simulink model "ng_pv_dynamic_dbus_p_4_ss_pmu"  (Simulink 8.8)
settings: Solver=ode4  StartTime=0.0  StopTime=inf  FixedStep=0.000125  RelTol=1e-3  EnableMultiTasking=on
PreLoadFcn:
  | Ts=125e-6;Core_Num = 0; np=1; nq=1; Vmin=.9;
PostLoadFcn:
  | Ts=125e-6;Core_Num = 0; np=1; nq=1; Vmin=.9;
InitFcn:
  | Ts=125e-6;Core_Num = 0; np=1; nq=1; Vmin=.9;
libraries: powerlib_meascontrol x180, rtio_generic_c37_118 x22, simulink x22, opal_lib x4, artemis x1, rtlab x1, powerlib x1
(part 2 of 4)

== system ng_pv_dynamic_dbus_p_4_ss_pmu/SS_PMU/Subsystem31 ==
  PMU in : Inport
  Bus Selector : BusSelector  OutputSignals=Measurements,FREQ,FROC
  Constant28 : Constant  Value=-1
  Constant29 : Constant  Value=-1
  Subsystem : Subsystem
  Phasors : Outport
  Analog : Outport  Port=2
  Ditigal : Outport  Port=3
  FREQ : Outport  Port=4
  FROC : Outport  Port=5
  wires:
  Subsystem/1(Out1) -> Bus Selector/1
  Bus Selector/1 -> Phasors/1  "<Measurements>"
  PMU in/1 -> Subsystem/1(In1)
  Constant28/1 -> Analog/1
  Constant29/1 -> Ditigal/1
  Bus Selector/2 -> FREQ/1  "<FREQ>"
  Bus Selector/3 -> FROC/1  "<FROC>"

== system ng_pv_dynamic_dbus_p_4_ss_pmu/SS_PMU/Subsystem32 ==
  PMU in : Inport
  Bus Selector : BusSelector  OutputSignals=Measurements,FREQ,FROC
  Constant28 : Constant  Value=-1
  Constant29 : Constant  Value=-1
  Subsystem : Subsystem
  Phasors : Outport
  Analog : Outport  Port=2
  Ditigal : Outport  Port=3
  FREQ : Outport  Port=4
  FROC : Outport  Port=5
  wires:
  Subsystem/1(Out1) -> Bus Selector/1
  Bus Selector/1 -> Phasors/1  "<Measurements>"
  PMU in/1 -> Subsystem/1(In1)
  Constant28/1 -> Analog/1
  Constant29/1 -> Ditigal/1
  Bus Selector/2 -> FREQ/1  "<FREQ>"
  Bus Selector/3 -> FROC/1  "<FROC>"

== system ng_pv_dynamic_dbus_p_4_ss_pmu/SS_PMU/Subsystem33 ==
  PMU in : Inport
  Bus Selector : BusSelector  OutputSignals=Measurements,FREQ,FROC
  Constant28 : Constant  Value=-1
  Constant29 : Constant  Value=-1
  Subsystem : Subsystem
  Phasors : Outport
  Analog : Outport  Port=2
  Ditigal : Outport  Port=3
  FREQ : Outport  Port=4
  FROC : Outport  Port=5
  wires:
  Subsystem/1(Out1) -> Bus Selector/1
  Bus Selector/1 -> Phasors/1  "<Measurements>"
  PMU in/1 -> Subsystem/1(In1)
  Constant28/1 -> Analog/1
  Constant29/1 -> Ditigal/1
  Bus Selector/2 -> FREQ/1  "<FREQ>"
  Bus Selector/3 -> FROC/1  "<FROC>"

== system ng_pv_dynamic_dbus_p_4_ss_pmu/SS_PMU/Subsystem34 ==
  PMU in : Inport
  Bus Selector : BusSelector  OutputSignals=Measurements,FREQ,FROC
  Constant28 : Constant  Value=-1
  Constant29 : Constant  Value=-1
  Subsystem : Subsystem
  Phasors : Outport
  Analog : Outport  Port=2
  Ditigal : Outport  Port=3
  FREQ : Outport  Port=4
  FROC : Outport  Port=5
  wires:
  Subsystem/1(Out1) -> Bus Selector/1
  Bus Selector/1 -> Phasors/1  "<Measurements>"
  PMU in/1 -> Subsystem/1(In1)
  Constant28/1 -> Analog/1
  Constant29/1 -> Ditigal/1
  Bus Selector/2 -> FREQ/1  "<FREQ>"
  Bus Selector/3 -> FROC/1  "<FROC>"

== system ng_pv_dynamic_dbus_p_4_ss_pmu/SS_PMU/Subsystem35 ==
  PMU in : Inport
  Bus Selector : BusSelector  OutputSignals=Measurements,FREQ,FROC
  Constant28 : Constant  Value=-1
  Constant29 : Constant  Value=-1
  Subsystem : Subsystem
  Phasors : Outport
  Analog : Outport  Port=2
  Ditigal : Outport  Port=3
  FREQ : Outport  Port=4
  FROC : Outport  Port=5
  wires:
  Subsystem/1(Out1) -> Bus Selector/1
  Bus Selector/1 -> Phasors/1  "<Measurements>"
  PMU in/1 -> Subsystem/1(In1)
  Constant28/1 -> Analog/1
  Constant29/1 -> Ditigal/1
  Bus Selector/2 -> FREQ/1  "<FREQ>"
  Bus Selector/3 -> FROC/1  "<FROC>"

== system ng_pv_dynamic_dbus_p_4_ss_pmu/SS_PMU/Subsystem36 ==
  PMU in : Inport
  Bus Selector : BusSelector  OutputSignals=Measurements,FREQ,FROC
  Constant28 : Constant  Value=-1
  Constant29 : Constant  Value=-1
  Subsystem : Subsystem
  Phasors : Outport
  Analog : Outport  Port=2
  Ditigal : Outport  Port=3
  FREQ : Outport  Port=4
  FROC : Outport  Port=5
  wires:
  Subsystem/1(Out1) -> Bus Selector/1
  Bus Selector/1 -> Phasors/1  "<Measurements>"
  PMU in/1 -> Subsystem/1(In1)
  Constant28/1 -> Analog/1
  Constant29/1 -> Ditigal/1
  Bus Selector/2 -> FREQ/1  "<FREQ>"
  Bus Selector/3 -> FROC/1  "<FROC>"

== system ng_pv_dynamic_dbus_p_4_ss_pmu/SS_PMU/Subsystem37 ==
  PMU in : Inport
  Bus Selector : BusSelector  OutputSignals=Measurements,FREQ,FROC
  Constant28 : Constant  Value=-1
  Constant29 : Constant  Value=-1
  Subsystem : Subsystem
  Phasors : Outport
  Analog : Outport  Port=2
  Ditigal : Outport  Port=3
  FREQ : Outport  Port=4
  FROC : Outport  Port=5
  wires:
  Subsystem/1(Out1) -> Bus Selector/1
  Bus Selector/1 -> Phasors/1  "<Measurements>"
  PMU in/1 -> Subsystem/1(In1)
  Constant28/1 -> Analog/1
  Constant29/1 -> Ditigal/1
  Bus Selector/2 -> FREQ/1  "<FREQ>"
  Bus Selector/3 -> FROC/1  "<FROC>"

== system ng_pv_dynamic_dbus_p_4_ss_pmu/SS_PMU/Subsystem38 ==
  PMU in : Inport
  Bus Selector : BusSelector  OutputSignals=Measurements,FREQ,FROC
  Constant28 : Constant  Value=-1
  Constant29 : Constant  Value=-1
  Subsystem : Subsystem
  Phasors : Outport
  Analog : Outport  Port=2
  Ditigal : Outport  Port=3
  FREQ : Outport  Port=4
  FROC : Outport  Port=5
  wires:
  Subsystem/1(Out1) -> Bus Selector/1
  Bus Selector/1 -> Phasors/1  "<Measurements>"
  PMU in/1 -> Subsystem/1(In1)
  Constant28/1 -> Analog/1
  Constant29/1 -> Ditigal/1
  Bus Selector/2 -> FREQ/1  "<FREQ>"
  Bus Selector/3 -> FROC/1  "<FROC>"

== system ng_pv_dynamic_dbus_p_4_ss_pmu/SS_PMU/Subsystem39 ==
  PMU in : Inport
  Bus Selector : BusSelector  OutputSignals=Measurements,FREQ,FROC
  Constant28 : Constant  Value=-1
  Constant29 : Constant  Value=-1
  Subsystem : Subsystem
  Phasors : Outport
  Analog : Outport  Port=2
  Ditigal : Outport  Port=3
  FREQ : Outport  Port=4
  FROC : Outport  Port=5
  wires:
  Subsystem/1(Out1) -> Bus Selector/1
  Bus Selector/1 -> Phasors/1  "<Measurements>"
  PMU in/1 -> Subsystem/1(In1)
  Constant28/1 -> Analog/1
  Constant29/1 -> Ditigal/1
  Bus Selector/2 -> FREQ/1  "<FREQ>"
  Bus Selector/3 -> FROC/1  "<FROC>"

== system ng_pv_dynamic_dbus_p_4_ss_pmu/SS_PMU/Subsystem4 ==
  Measurements : Inport
  Demux7 : Demux  Outputs=6
  Demux8 : Demux  Outputs=6
  Mux5 : Mux  Inputs=12
  Subsystem : Subsystem
  Phasors : Outport
  Phasor_Freq : Outport  Port=2
  FROC : Outport  Port=3
  wires:
  Mux5/1 -> Phasors/1
  Demux7/4 -> [Phase_Va]
  Demux7/1 -> [Mag_Va]
  Demux7/2 -> [Mag_Vb]
  Demux7/3 -> [Mag_Vc]
  Subsystem/1(Phasors_Vabc) -> Demux7/1
  Demux7/6 -> [Phase_Vc]
  Demux7/5 -> [Phase_Vb]
  Subsystem/3(Phasor_Freq) -> Phasor_Freq/1
  Measurements/1 -> Subsystem/1(Measurements1)
  Subsystem/4(Phasor_DTFreq) -> FROC/1
  Demux8/2 -> [Mag_Ib]
  Demux8/4 -> [Phase_Ia]
  Demux8/5 -> [Phase_Ib]
  Subsystem/2(Phasors_Iabc) -> Demux8/1
  Demux8/3 -> [Mag_Ic]
  Demux8/1 -> [Mag_Ia]
  Demux8/6 -> [Phase_Ic]
  [Phase_Ic] -> Mux5/12
  [Mag_Ic] -> Mux5/11
  [Phase_Ib] -> Mux5/10
  [Mag_Ib] -> Mux5/9
  [Phase_Ia] -> Mux5/8
  [Mag_Ia] -> Mux5/7
  [Phase_Vc] -> Mux5/6
  [Mag_Vc] -> Mux5/5
  [Phase_Vb] -> Mux5/4
  [Mag_Vb] -> Mux5/3
  [Phase_Va] -> Mux5/2
  [Mag_Va] -> Mux5/1

== system ng_pv_dynamic_dbus_p_4_ss_pmu/SS_PMU/Subsystem40 ==
  PMU in : Inport
  Bus Selector : BusSelector  OutputSignals=Measurements,FREQ,FROC
  Constant28 : Constant  Value=-1
  Constant29 : Constant  Value=-1
  Subsystem : Subsystem
  Phasors : Outport
  Analog : Outport  Port=2
  Ditigal : Outport  Port=3
  FREQ : Outport  Port=4
  FROC : Outport  Port=5
  wires:
  Subsystem/1(Out1) -> Bus Selector/1
  Bus Selector/1 -> Phasors/1  "<Measurements>"
  PMU in/1 -> Subsystem/1(In1)
  Constant28/1 -> Analog/1
  Constant29/1 -> Ditigal/1
  Bus Selector/2 -> FREQ/1  "<FREQ>"
  Bus Selector/3 -> FROC/1  "<FROC>"

== system ng_pv_dynamic_dbus_p_4_ss_pmu/SS_PMU/Subsystem41 ==
  PMU in : Inport
  Bus Selector : BusSelector  OutputSignals=Measurements,FREQ,FROC
  Constant28 : Constant  Value=-1
  Constant29 : Constant  Value=-1
  Subsystem : Subsystem
  Phasors : Outport
  Analog : Outport  Port=2
  Ditigal : Outport  Port=3
  FREQ : Outport  Port=4
  FROC : Outport  Port=5
  wires:
  Subsystem/1(Out1) -> Bus Selector/1
  Bus Selector/1 -> Phasors/1  "<Measurements>"
  PMU in/1 -> Subsystem/1(In1)
  Constant28/1 -> Analog/1
  Constant29/1 -> Ditigal/1
  Bus Selector/2 -> FREQ/1  "<FREQ>"
  Bus Selector/3 -> FROC/1  "<FROC>"

== system ng_pv_dynamic_dbus_p_4_ss_pmu/SS_PMU/Subsystem42 ==
  PMU in : Inport
  Bus Selector : BusSelector  OutputSignals=Measurements,FREQ,FROC
  Constant28 : Constant  Value=-1
  Constant29 : Constant  Value=-1
  Subsystem : Subsystem
  Phasors : Outport
  Analog : Outport  Port=2
  Ditigal : Outport  Port=3
  FREQ : Outport  Port=4
  FROC : Outport  Port=5
  wires:
  Subsystem/1(Out1) -> Bus Selector/1
  Bus Selector/1 -> Phasors/1  "<Measurements>"
  PMU in/1 -> Subsystem/1(In1)
  Constant28/1 -> Analog/1
  Constant29/1 -> Ditigal/1
  Bus Selector/2 -> FREQ/1  "<FREQ>"
  Bus Selector/3 -> FROC/1  "<FROC>"

== system ng_pv_dynamic_dbus_p_4_ss_pmu/SS_PMU/Subsystem43 ==
  PMU in : Inport
  Bus Selector : BusSelector  OutputSignals=Measurements,FREQ,FROC
  Constant28 : Constant  Value=-1
  Constant29 : Constant  Value=-1
  Subsystem : Subsystem
  Phasors : Outport
  Analog : Outport  Port=2
  Ditigal : Outport  Port=3
  FREQ : Outport  Port=4
  FROC : Outport  Port=5
  wires:
  Subsystem/1(Out1) -> Bus Selector/1
  Bus Selector/1 -> Phasors/1  "<Measurements>"
  PMU in/1 -> Subsystem/1(In1)
  Constant28/1 -> Analog/1
  Constant29/1 -> Ditigal/1
  Bus Selector/2 -> FREQ/1  "<FREQ>"
  Bus Selector/3 -> FROC/1  "<FROC>"

== system ng_pv_dynamic_dbus_p_4_ss_pmu/SS_PMU/Subsystem44 ==
  PMU in : Inport
  Bus Selector : BusSelector  OutputSignals=Measurements,FREQ,FROC
  Constant28 : Constant  Value=-1
  Constant29 : Constant  Value=-1
  Subsystem : Subsystem
  Phasors : Outport
  Analog : Outport  Port=2
  Ditigal : Outport  Port=3
  FREQ : Outport  Port=4
  FROC : Outport  Port=5
  wires:
  Subsystem/1(Out1) -> Bus Selector/1
  Bus Selector/1 -> Phasors/1  "<Measurements>"
  PMU in/1 -> Subsystem/1(In1)
  Constant28/1 -> Analog/1
  Constant29/1 -> Ditigal/1
  Bus Selector/2 -> FREQ/1  "<FREQ>"
  Bus Selector/3 -> FROC/1  "<FROC>"

== system ng_pv_dynamic_dbus_p_4_ss_pmu/SS_PMU/Subsystem5 ==
  Measurements : Inport
  Demux7 : Demux  Outputs=6
  Demux8 : Demux  Outputs=6
  Mux5 : Mux  Inputs=12
  Subsystem : Subsystem
  Phasors : Outport
  Phasor_Freq : Outport  Port=2
  FROC : Outport  Port=3
  wires:
  Mux5/1 -> Phasors/1
  Demux7/4 -> [Phase_Va]
  Demux7/1 -> [Mag_Va]
  Demux7/2 -> [Mag_Vb]
  Demux7/3 -> [Mag_Vc]
  Subsystem/1(Phasors_Vabc) -> Demux7/1
  Demux7/6 -> [Phase_Vc]
  Demux7/5 -> [Phase_Vb]
  Subsystem/3(Phasor_Freq) -> Phasor_Freq/1
  Measurements/1 -> Subsystem/1(Measurements1)
  Subsystem/4(Phasor_DTFreq) -> FROC/1
  Demux8/2 -> [Mag_Ib]
  Demux8/4 -> [Phase_Ia]
  Demux8/5 -> [Phase_Ib]
  Subsystem/2(Phasors_Iabc) -> Demux8/1
  Demux8/3 -> [Mag_Ic]
  Demux8/1 -> [Mag_Ia]
  Demux8/6 -> [Phase_Ic]
  [Phase_Ic] -> Mux5/12
  [Mag_Ic] -> Mux5/11
  [Phase_Ib] -> Mux5/10
  [Mag_Ib] -> Mux5/9
  [Phase_Ia] -> Mux5/8
  [Mag_Ia] -> Mux5/7
  [Phase_Vc] -> Mux5/6
  [Mag_Vc] -> Mux5/5
  [Phase_Vb] -> Mux5/4
  [Mag_Vb] -> Mux5/3
  [Phase_Va] -> Mux5/2
  [Mag_Va] -> Mux5/1

== system ng_pv_dynamic_dbus_p_4_ss_pmu/SS_PMU/Subsystem6 ==
  Measurements : Inport
  Demux7 : Demux  Outputs=6
  Demux8 : Demux  Outputs=6
  Mux5 : Mux  Inputs=12
  Subsystem : Subsystem
  Phasors : Outport
  Phasor_Freq : Outport  Port=2
  FROC : Outport  Port=3
  wires:
  Mux5/1 -> Phasors/1
  Demux7/4 -> [Phase_Va]
  Demux7/1 -> [Mag_Va]
  Demux7/2 -> [Mag_Vb]
  Demux7/3 -> [Mag_Vc]
  Subsystem/1(Phasors_Vabc) -> Demux7/1
  Demux7/6 -> [Phase_Vc]
  Demux7/5 -> [Phase_Vb]
  Subsystem/3(Phasor_Freq) -> Phasor_Freq/1
  Measurements/1 -> Subsystem/1(Measurements1)
  Subsystem/4(Phasor_DTFreq) -> FROC/1
  Demux8/2 -> [Mag_Ib]
  Demux8/4 -> [Phase_Ia]
  Demux8/5 -> [Phase_Ib]
  Subsystem/2(Phasors_Iabc) -> Demux8/1
  Demux8/3 -> [Mag_Ic]
  Demux8/1 -> [Mag_Ia]
  Demux8/6 -> [Phase_Ic]
  [Phase_Ic] -> Mux5/12
  [Mag_Ic] -> Mux5/11
  [Phase_Ib] -> Mux5/10
  [Mag_Ib] -> Mux5/9
  [Phase_Ia] -> Mux5/8
  [Mag_Ia] -> Mux5/7
  [Phase_Vc] -> Mux5/6
  [Mag_Vc] -> Mux5/5
  [Phase_Vb] -> Mux5/4
  [Mag_Vb] -> Mux5/3
  [Phase_Va] -> Mux5/2
  [Mag_Va] -> Mux5/1

== system ng_pv_dynamic_dbus_p_4_ss_pmu/SS_PMU/Subsystem7 ==
  Measurements : Inport
  Demux7 : Demux  Outputs=6
  Demux8 : Demux  Outputs=6
  Mux5 : Mux  Inputs=12
  Subsystem : Subsystem
  Phasors : Outport
  Phasor_Freq : Outport  Port=2
  FROC : Outport  Port=3
  wires:
  Mux5/1 -> Phasors/1
  Demux7/4 -> [Phase_Va]
  Demux7/1 -> [Mag_Va]
  Demux7/2 -> [Mag_Vb]
  Demux7/3 -> [Mag_Vc]
  Subsystem/1(Phasors_Vabc) -> Demux7/1
  Demux7/6 -> [Phase_Vc]
  Demux7/5 -> [Phase_Vb]
  Subsystem/3(Phasor_Freq) -> Phasor_Freq/1
  Measurements/1 -> Subsystem/1(Measurements1)
  Subsystem/4(Phasor_DTFreq) -> FROC/1
  Demux8/2 -> [Mag_Ib]
  Demux8/4 -> [Phase_Ia]
  Demux8/5 -> [Phase_Ib]
  Subsystem/2(Phasors_Iabc) -> Demux8/1
  Demux8/3 -> [Mag_Ic]
  Demux8/1 -> [Mag_Ia]
  Demux8/6 -> [Phase_Ic]
  [Phase_Ic] -> Mux5/12
  [Mag_Ic] -> Mux5/11
  [Phase_Ib] -> Mux5/10
  [Mag_Ib] -> Mux5/9
  [Phase_Ia] -> Mux5/8
  [Mag_Ia] -> Mux5/7
  [Phase_Vc] -> Mux5/6
  [Mag_Vc] -> Mux5/5
  [Phase_Vb] -> Mux5/4
  [Mag_Vb] -> Mux5/3
  [Phase_Va] -> Mux5/2
  [Mag_Va] -> Mux5/1

== system ng_pv_dynamic_dbus_p_4_ss_pmu/SS_PMU/Subsystem8 ==
  Measurements : Inport
  Demux7 : Demux  Outputs=6
  Demux8 : Demux  Outputs=6
  Mux5 : Mux  Inputs=12
  Subsystem : Subsystem
  Phasors : Outport
  Phasor_Freq : Outport  Port=2
  FROC : Outport  Port=3
  wires:
  Mux5/1 -> Phasors/1
  Demux7/4 -> [Phase_Va]
  Demux7/1 -> [Mag_Va]
  Demux7/2 -> [Mag_Vb]
  Demux7/3 -> [Mag_Vc]
  Subsystem/1(Phasors_Vabc) -> Demux7/1
  Demux7/6 -> [Phase_Vc]
  Demux7/5 -> [Phase_Vb]
  Subsystem/3(Phasor_Freq) -> Phasor_Freq/1
  Measurements/1 -> Subsystem/1(Measurements1)
  Subsystem/4(Phasor_DTFreq) -> FROC/1
  Demux8/2 -> [Mag_Ib]
  Demux8/4 -> [Phase_Ia]
  Demux8/5 -> [Phase_Ib]
  Subsystem/2(Phasors_Iabc) -> Demux8/1
  Demux8/3 -> [Mag_Ic]
  Demux8/1 -> [Mag_Ia]
  Demux8/6 -> [Phase_Ic]
  [Phase_Ic] -> Mux5/12
  [Mag_Ic] -> Mux5/11
  [Phase_Ib] -> Mux5/10
  [Mag_Ib] -> Mux5/9
  [Phase_Ia] -> Mux5/8
  [Mag_Ia] -> Mux5/7
  [Phase_Vc] -> Mux5/6
  [Mag_Vc] -> Mux5/5
  [Phase_Vb] -> Mux5/4
  [Mag_Vb] -> Mux5/3
  [Phase_Va] -> Mux5/2
  [Mag_Va] -> Mux5/1

== system ng_pv_dynamic_dbus_p_4_ss_pmu/SS_PMU/Subsystem9 ==
  Measurements : Inport
  Demux7 : Demux  Outputs=6
  Demux8 : Demux  Outputs=6
  Mux5 : Mux  Inputs=12
  Subsystem : Subsystem
  Phasors : Outport
  Phasor_Freq : Outport  Port=2
  FROC : Outport  Port=3
  wires:
  Mux5/1 -> Phasors/1
  Demux7/4 -> [Phase_Va]
  Demux7/1 -> [Mag_Va]
  Demux7/2 -> [Mag_Vb]
  Demux7/3 -> [Mag_Vc]
  Subsystem/1(Phasors_Vabc) -> Demux7/1
  Demux7/6 -> [Phase_Vc]
  Demux7/5 -> [Phase_Vb]
  Subsystem/3(Phasor_Freq) -> Phasor_Freq/1
  Measurements/1 -> Subsystem/1(Measurements1)
  Subsystem/4(Phasor_DTFreq) -> FROC/1
  Demux8/2 -> [Mag_Ib]
  Demux8/4 -> [Phase_Ia]
  Demux8/5 -> [Phase_Ib]
  Subsystem/2(Phasors_Iabc) -> Demux8/1
  Demux8/3 -> [Mag_Ic]
  Demux8/1 -> [Mag_Ia]
  Demux8/6 -> [Phase_Ic]
  [Phase_Ic] -> Mux5/12
  [Mag_Ic] -> Mux5/11
  [Phase_Ib] -> Mux5/10
  [Mag_Ib] -> Mux5/9
  [Phase_Ia] -> Mux5/8
  [Mag_Ia] -> Mux5/7
  [Phase_Vc] -> Mux5/6
  [Mag_Vc] -> Mux5/5
  [Phase_Vb] -> Mux5/4
  [Mag_Vb] -> Mux5/3
  [Phase_Va] -> Mux5/2
  [Mag_Va] -> Mux5/1

== system ng_pv_dynamic_dbus_p_4_ss_pmu/SS_PMU/rtlab_send_subsystem ==
  Subsystem1 : Subsystem
  wires:
  [rtlab_send_1] -> Subsystem1/1(In1)

== system ng_pv_dynamic_dbus_p_4_ss_pmu/SS_PMU/zzzOpComm ==
  Demux_1 : Demux  Outputs="[120    3]"
  Demux_2 : Demux  Outputs=[62]
  Receive_1 : opal_lib/Communication/OpRec_rt  src=1  Data_width=123  st=0.000125
  Receive_2 : opal_lib/Communication/OpRec_rt  src=3  Data_width=62  st=0.000125
  busStruct : Subsystem
  Out1 : Outport
  Out2 : Outport  Port=2
  Out3 : Outport  Port=3
  wires:
  Demux_2/1 -> busStruct/3(In3)
  Demux_1/2 -> busStruct/2(In2)
  Demux_1/1 -> busStruct/1(In1)
  busStruct/3(Out3) -> Out3/1
  busStruct/2(Out2) -> Out2/1
  busStruct/1(Out1) -> Out1/1
  Receive_2/1 -> Demux_2/1
  Receive_1/1 -> Demux_1/1

== system ng_pv_dynamic_dbus_p_4_ss_pmu/SS_PMU/Subsystem1/Subsystem ==
  Measurements1 : Inport
  Demux7 : Demux  Outputs=2
  Subsystem1 : Subsystem
  Phasors_Vabc : Outport
  Phasors_Iabc : Outport  Port=2
  Phasor_Freq : Outport  Port=3
  Phasor_DTFreq : Outport  Port=4
  wires:
  Measurements1/1 -> Subsystem1/1(Measurements)
  Subsystem1/2(Phasors_Freq) -> Phasor_Freq/1
  Subsystem1/3(Phasors_DTFreq) -> Phasor_DTFreq/1
  Demux7/2 -> Phasors_Iabc/1
  Demux7/1 -> Phasors_Vabc/1
  Subsystem1/1(Phasors_abc) -> Demux7/1

== system ng_pv_dynamic_dbus_p_4_ss_pmu/SS_PMU/Subsystem10/Subsystem ==
  Measurements1 : Inport
  Demux7 : Demux  Outputs=2
  Subsystem1 : Subsystem
  Phasors_Vabc : Outport
  Phasors_Iabc : Outport  Port=2
  Phasor_Freq : Outport  Port=3
  Phasor_DTFreq : Outport  Port=4
  wires:
  Measurements1/1 -> Subsystem1/1(Measurements)
  Subsystem1/2(Phasors_Freq) -> Phasor_Freq/1
  Subsystem1/3(Phasors_DTFreq) -> Phasor_DTFreq/1
  Demux7/2 -> Phasors_Iabc/1
  Demux7/1 -> Phasors_Vabc/1
  Subsystem1/1(Phasors_abc) -> Demux7/1

== system ng_pv_dynamic_dbus_p_4_ss_pmu/SS_PMU/Subsystem11/Subsystem ==
  Measurements1 : Inport
  Demux7 : Demux  Outputs=2
  Subsystem1 : Subsystem
  Phasors_Vabc : Outport
  Phasors_Iabc : Outport  Port=2
  Phasor_Freq : Outport  Port=3
  Phasor_DTFreq : Outport  Port=4
  wires:
  Measurements1/1 -> Subsystem1/1(Measurements)
  Subsystem1/2(Phasors_Freq) -> Phasor_Freq/1
  Subsystem1/3(Phasors_DTFreq) -> Phasor_DTFreq/1
  Demux7/2 -> Phasors_Iabc/1
  Demux7/1 -> Phasors_Vabc/1
  Subsystem1/1(Phasors_abc) -> Demux7/1

== system ng_pv_dynamic_dbus_p_4_ss_pmu/SS_PMU/Subsystem12/Subsystem ==
  Measurements1 : Inport
  Demux7 : Demux  Outputs=2
  Subsystem1 : Subsystem
  Phasors_Vabc : Outport
  Phasors_Iabc : Outport  Port=2
  Phasor_Freq : Outport  Port=3
  Phasor_DTFreq : Outport  Port=4
  wires:
  Measurements1/1 -> Subsystem1/1(Measurements)
  Subsystem1/2(Phasors_Freq) -> Phasor_Freq/1
  Subsystem1/3(Phasors_DTFreq) -> Phasor_DTFreq/1
  Demux7/2 -> Phasors_Iabc/1
  Demux7/1 -> Phasors_Vabc/1
  Subsystem1/1(Phasors_abc) -> Demux7/1

== system ng_pv_dynamic_dbus_p_4_ss_pmu/SS_PMU/Subsystem13/Subsystem ==
  Measurements1 : Inport
  Demux7 : Demux  Outputs=2
  Subsystem1 : Subsystem
  Phasors_Vabc : Outport
  Phasors_Iabc : Outport  Port=2
  Phasor_Freq : Outport  Port=3
  Phasor_DTFreq : Outport  Port=4
  wires:
  Measurements1/1 -> Subsystem1/1(Measurements)
  Subsystem1/2(Phasors_Freq) -> Phasor_Freq/1
  Subsystem1/3(Phasors_DTFreq) -> Phasor_DTFreq/1
  Demux7/2 -> Phasors_Iabc/1
  Demux7/1 -> Phasors_Vabc/1
  Subsystem1/1(Phasors_abc) -> Demux7/1

== system ng_pv_dynamic_dbus_p_4_ss_pmu/SS_PMU/Subsystem14/Subsystem ==
  Measurements1 : Inport
  Demux7 : Demux  Outputs=2
  Subsystem1 : Subsystem
  Phasors_Vabc : Outport
  Phasors_Iabc : Outport  Port=2
  Phasor_Freq : Outport  Port=3
  Phasor_DTFreq : Outport  Port=4
  wires:
  Measurements1/1 -> Subsystem1/1(Measurements)
  Subsystem1/2(Phasors_Freq) -> Phasor_Freq/1
  Subsystem1/3(Phasors_DTFreq) -> Phasor_DTFreq/1
  Demux7/2 -> Phasors_Iabc/1
  Demux7/1 -> Phasors_Vabc/1
  Subsystem1/1(Phasors_abc) -> Demux7/1

== system ng_pv_dynamic_dbus_p_4_ss_pmu/SS_PMU/Subsystem15/Subsystem ==
  Measurements1 : Inport
  Demux7 : Demux  Outputs=2
  Subsystem1 : Subsystem
  Phasors_Vabc : Outport
  Phasors_Iabc : Outport  Port=2
  Phasor_Freq : Outport  Port=3
  Phasor_DTFreq : Outport  Port=4
  wires:
  Measurements1/1 -> Subsystem1/1(Measurements)
  Subsystem1/2(Phasors_Freq) -> Phasor_Freq/1
  Subsystem1/3(Phasors_DTFreq) -> Phasor_DTFreq/1
  Demux7/2 -> Phasors_Iabc/1
  Demux7/1 -> Phasors_Vabc/1
  Subsystem1/1(Phasors_abc) -> Demux7/1

== system ng_pv_dynamic_dbus_p_4_ss_pmu/SS_PMU/Subsystem16/Subsystem ==
  Measurements1 : Inport
  Demux7 : Demux  Outputs=2
  Subsystem1 : Subsystem
  Phasors_Vabc : Outport
  Phasors_Iabc : Outport  Port=2
  Phasor_Freq : Outport  Port=3
  Phasor_DTFreq : Outport  Port=4
  wires:
  Measurements1/1 -> Subsystem1/1(Measurements)
  Subsystem1/2(Phasors_Freq) -> Phasor_Freq/1
  Subsystem1/3(Phasors_DTFreq) -> Phasor_DTFreq/1
  Demux7/2 -> Phasors_Iabc/1
  Demux7/1 -> Phasors_Vabc/1
  Subsystem1/1(Phasors_abc) -> Demux7/1

== system ng_pv_dynamic_dbus_p_4_ss_pmu/SS_PMU/Subsystem17/Subsystem ==
  Measurements1 : Inport
  Demux7 : Demux  Outputs=2
  Subsystem1 : Subsystem
  Phasors_Vabc : Outport
  Phasors_Iabc : Outport  Port=2
  Phasor_Freq : Outport  Port=3
  Phasor_DTFreq : Outport  Port=4
  wires:
  Measurements1/1 -> Subsystem1/1(Measurements)
  Subsystem1/2(Phasors_Freq) -> Phasor_Freq/1
  Subsystem1/3(Phasors_DTFreq) -> Phasor_DTFreq/1
  Demux7/2 -> Phasors_Iabc/1
  Demux7/1 -> Phasors_Vabc/1
  Subsystem1/1(Phasors_abc) -> Demux7/1

== system ng_pv_dynamic_dbus_p_4_ss_pmu/SS_PMU/Subsystem18/Subsystem ==
  Measurements1 : Inport
  Demux7 : Demux  Outputs=2
  Subsystem1 : Subsystem
  Phasors_Vabc : Outport
  Phasors_Iabc : Outport  Port=2
  Phasor_Freq : Outport  Port=3
  Phasor_DTFreq : Outport  Port=4
  wires:
  Measurements1/1 -> Subsystem1/1(Measurements)
  Subsystem1/2(Phasors_Freq) -> Phasor_Freq/1
  Subsystem1/3(Phasors_DTFreq) -> Phasor_DTFreq/1
  Demux7/2 -> Phasors_Iabc/1
  Demux7/1 -> Phasors_Vabc/1
  Subsystem1/1(Phasors_abc) -> Demux7/1

== system ng_pv_dynamic_dbus_p_4_ss_pmu/SS_PMU/Subsystem19/Subsystem ==
  Measurements1 : Inport
  Demux7 : Demux  Outputs=2
  Subsystem1 : Subsystem
  Phasors_Vabc : Outport
  Phasors_Iabc : Outport  Port=2
  Phasor_Freq : Outport  Port=3
  Phasor_DTFreq : Outport  Port=4
  wires:
  Measurements1/1 -> Subsystem1/1(Measurements)
  Subsystem1/2(Phasors_Freq) -> Phasor_Freq/1
  Subsystem1/3(Phasors_DTFreq) -> Phasor_DTFreq/1
  Demux7/2 -> Phasors_Iabc/1
  Demux7/1 -> Phasors_Vabc/1
  Subsystem1/1(Phasors_abc) -> Demux7/1

== system ng_pv_dynamic_dbus_p_4_ss_pmu/SS_PMU/Subsystem2/Subsystem ==
  Measurements1 : Inport
  Demux7 : Demux  Outputs=2
  Subsystem1 : Subsystem
  Phasors_Vabc : Outport
  Phasors_Iabc : Outport  Port=2
  Phasor_Freq : Outport  Port=3
  Phasor_DTFreq : Outport  Port=4
  wires:
  Measurements1/1 -> Subsystem1/1(Measurements)
  Subsystem1/2(Phasors_Freq) -> Phasor_Freq/1
  Subsystem1/3(Phasors_DTFreq) -> Phasor_DTFreq/1
  Demux7/2 -> Phasors_Iabc/1
  Demux7/1 -> Phasors_Vabc/1
  Subsystem1/1(Phasors_abc) -> Demux7/1

== system ng_pv_dynamic_dbus_p_4_ss_pmu/SS_PMU/Subsystem20/Subsystem ==
  Measurements1 : Inport
  Demux7 : Demux  Outputs=2
  Subsystem1 : Subsystem
  Phasors_Vabc : Outport
  Phasors_Iabc : Outport  Port=2
  Phasor_Freq : Outport  Port=3
  Phasor_DTFreq : Outport  Port=4
  wires:
  Measurements1/1 -> Subsystem1/1(Measurements)
  Subsystem1/2(Phasors_Freq) -> Phasor_Freq/1
  Subsystem1/3(Phasors_DTFreq) -> Phasor_DTFreq/1
  Demux7/2 -> Phasors_Iabc/1
  Demux7/1 -> Phasors_Vabc/1
  Subsystem1/1(Phasors_abc) -> Demux7/1

== system ng_pv_dynamic_dbus_p_4_ss_pmu/SS_PMU/Subsystem21/Subsystem ==
  Measurements1 : Inport
  Demux7 : Demux  Outputs=2
  Subsystem1 : Subsystem
  Phasors_Vabc : Outport
  Phasors_Iabc : Outport  Port=2
  Phasor_Freq : Outport  Port=3
  Phasor_DTFreq : Outport  Port=4
  wires:
  Measurements1/1 -> Subsystem1/1(Measurements)
  Subsystem1/2(Phasors_Freq) -> Phasor_Freq/1
  Subsystem1/3(Phasors_DTFreq) -> Phasor_DTFreq/1
  Demux7/2 -> Phasors_Iabc/1
  Demux7/1 -> Phasors_Vabc/1
  Subsystem1/1(Phasors_abc) -> Demux7/1

== system ng_pv_dynamic_dbus_p_4_ss_pmu/SS_PMU/Subsystem22/Subsystem ==
  Measurements1 : Inport
  Demux7 : Demux  Outputs=2
  Subsystem1 : Subsystem
  Phasors_Vabc : Outport
  Phasors_Iabc : Outport  Port=2
  Phasor_Freq : Outport  Port=3
  Phasor_DTFreq : Outport  Port=4
  wires:
  Measurements1/1 -> Subsystem1/1(Measurements)
  Subsystem1/2(Phasors_Freq) -> Phasor_Freq/1
  Subsystem1/3(Phasors_DTFreq) -> Phasor_DTFreq/1
  Demux7/2 -> Phasors_Iabc/1
  Demux7/1 -> Phasors_Vabc/1
  Subsystem1/1(Phasors_abc) -> Demux7/1

== system ng_pv_dynamic_dbus_p_4_ss_pmu/SS_PMU/Subsystem23/Subsystem ==
  In1 : Inport
  Bus Creator : BusCreator  Inputs=3
  Selector1 : Selector  InputPortWidth=14  IndexOptions=Index vector (dialog)  Indices=[13]  OutputSizes=1
  Selector2 : Selector  InputPortWidth=14  IndexOptions=Index vector (dialog)  Indices=[14]  OutputSizes=1
  Selector5 : Selector  InputPortWidth=14  IndexOptions=Index vector (dialog)  Indices=[1 2 3 4 5 6 7 8 9 10 11 12]  OutputSizes=1
  Out1 : Outport
  wires:
  In1/1 -> Selector5/1, Selector2/1, Selector1/1
  Selector5/1 -> Bus Creator/1  "Measurements"
  Bus Creator/1 -> Out1/1
  Selector1/1 -> Bus Creator/2  "FREQ"
  Selector2/1 -> Bus Creator/3  "FROC"

== system ng_pv_dynamic_dbus_p_4_ss_pmu/SS_PMU/Subsystem24/Subsystem ==
  In1 : Inport
  Bus Creator : BusCreator  Inputs=3
  Selector1 : Selector  InputPortWidth=14  IndexOptions=Index vector (dialog)  Indices=[13]  OutputSizes=1
  Selector2 : Selector  InputPortWidth=14  IndexOptions=Index vector (dialog)  Indices=[14]  OutputSizes=1
  Selector5 : Selector  InputPortWidth=14  IndexOptions=Index vector (dialog)  Indices=[1 2 3 4 5 6 7 8 9 10 11 12]  OutputSizes=1
  Out1 : Outport
  wires:
  In1/1 -> Selector5/1, Selector2/1, Selector1/1
  Selector5/1 -> Bus Creator/1  "Measurements"
  Bus Creator/1 -> Out1/1
  Selector1/1 -> Bus Creator/2  "FREQ"
  Selector2/1 -> Bus Creator/3  "FROC"

== system ng_pv_dynamic_dbus_p_4_ss_pmu/SS_PMU/Subsystem25/Subsystem ==
  In1 : Inport
  Bus Creator : BusCreator  Inputs=3
  Selector1 : Selector  InputPortWidth=14  IndexOptions=Index vector (dialog)  Indices=[13]  OutputSizes=1
  Selector2 : Selector  InputPortWidth=14  IndexOptions=Index vector (dialog)  Indices=[14]  OutputSizes=1
  Selector5 : Selector  InputPortWidth=14  IndexOptions=Index vector (dialog)  Indices=[1 2 3 4 5 6 7 8 9 10 11 12]  OutputSizes=1
  Out1 : Outport
  wires:
  In1/1 -> Selector5/1, Selector2/1, Selector1/1
  Selector5/1 -> Bus Creator/1  "Measurements"
  Bus Creator/1 -> Out1/1
  Selector1/1 -> Bus Creator/2  "FREQ"
  Selector2/1 -> Bus Creator/3  "FROC"

== system ng_pv_dynamic_dbus_p_4_ss_pmu/SS_PMU/Subsystem26/Subsystem ==
  In1 : Inport
  Bus Creator : BusCreator  Inputs=3
  Selector1 : Selector  InputPortWidth=14  IndexOptions=Index vector (dialog)  Indices=[13]  OutputSizes=1
  Selector2 : Selector  InputPortWidth=14  IndexOptions=Index vector (dialog)  Indices=[14]  OutputSizes=1
  Selector5 : Selector  InputPortWidth=14  IndexOptions=Index vector (dialog)  Indices=[1 2 3 4 5 6 7 8 9 10 11 12]  OutputSizes=1
  Out1 : Outport
  wires:
  In1/1 -> Selector5/1, Selector2/1, Selector1/1
  Selector5/1 -> Bus Creator/1  "Measurements"
  Bus Creator/1 -> Out1/1
  Selector1/1 -> Bus Creator/2  "FREQ"
  Selector2/1 -> Bus Creator/3  "FROC"

== system ng_pv_dynamic_dbus_p_4_ss_pmu/SS_PMU/Subsystem27/Subsystem ==
  In1 : Inport
  Bus Creator : BusCreator  Inputs=3
  Selector1 : Selector  InputPortWidth=14  IndexOptions=Index vector (dialog)  Indices=[13]  OutputSizes=1
  Selector2 : Selector  InputPortWidth=14  IndexOptions=Index vector (dialog)  Indices=[14]  OutputSizes=1
  Selector5 : Selector  InputPortWidth=14  IndexOptions=Index vector (dialog)  Indices=[1 2 3 4 5 6 7 8 9 10 11 12]  OutputSizes=1
  Out1 : Outport
  wires:
  In1/1 -> Selector5/1, Selector2/1, Selector1/1
  Selector5/1 -> Bus Creator/1  "Measurements"
  Bus Creator/1 -> Out1/1
  Selector1/1 -> Bus Creator/2  "FREQ"
  Selector2/1 -> Bus Creator/3  "FROC"

== system ng_pv_dynamic_dbus_p_4_ss_pmu/SS_PMU/Subsystem28/Subsystem ==
  In1 : Inport
  Bus Creator : BusCreator  Inputs=3
  Selector1 : Selector  InputPortWidth=14  IndexOptions=Index vector (dialog)  Indices=[13]  OutputSizes=1
  Selector2 : Selector  InputPortWidth=14  IndexOptions=Index vector (dialog)  Indices=[14]  OutputSizes=1
  Selector5 : Selector  InputPortWidth=14  IndexOptions=Index vector (dialog)  Indices=[1 2 3 4 5 6 7 8 9 10 11 12]  OutputSizes=1
  Out1 : Outport
  wires:
  In1/1 -> Selector5/1, Selector2/1, Selector1/1
  Selector5/1 -> Bus Creator/1  "Measurements"
  Bus Creator/1 -> Out1/1
  Selector1/1 -> Bus Creator/2  "FREQ"
  Selector2/1 -> Bus Creator/3  "FROC"

== system ng_pv_dynamic_dbus_p_4_ss_pmu/SS_PMU/Subsystem29/Subsystem ==
  In1 : Inport
  Bus Creator : BusCreator  Inputs=3
  Selector1 : Selector  InputPortWidth=14  IndexOptions=Index vector (dialog)  Indices=[13]  OutputSizes=1
  Selector2 : Selector  InputPortWidth=14  IndexOptions=Index vector (dialog)  Indices=[14]  OutputSizes=1
  Selector5 : Selector  InputPortWidth=14  IndexOptions=Index vector (dialog)  Indices=[1 2 3 4 5 6 7 8 9 10 11 12]  OutputSizes=1
  Out1 : Outport
  wires:
  In1/1 -> Selector5/1, Selector2/1, Selector1/1
  Selector5/1 -> Bus Creator/1  "Measurements"
  Bus Creator/1 -> Out1/1
  Selector1/1 -> Bus Creator/2  "FREQ"
  Selector2/1 -> Bus Creator/3  "FROC"

== system ng_pv_dynamic_dbus_p_4_ss_pmu/SS_PMU/Subsystem3/Subsystem ==
  Measurements1 : Inport
  Demux7 : Demux  Outputs=2
  Subsystem1 : Subsystem
  Phasors_Vabc : Outport
  Phasors_Iabc : Outport  Port=2
  Phasor_Freq : Outport  Port=3
  Phasor_DTFreq : Outport  Port=4
  wires:
  Measurements1/1 -> Subsystem1/1(Measurements)
  Subsystem1/2(Phasors_Freq) -> Phasor_Freq/1
  Subsystem1/3(Phasors_DTFreq) -> Phasor_DTFreq/1
  Demux7/2 -> Phasors_Iabc/1
  Demux7/1 -> Phasors_Vabc/1
  Subsystem1/1(Phasors_abc) -> Demux7/1

== system ng_pv_dynamic_dbus_p_4_ss_pmu/SS_PMU/Subsystem30/Subsystem ==
  In1 : Inport
  Bus Creator : BusCreator  Inputs=3
  Selector1 : Selector  InputPortWidth=14  IndexOptions=Index vector (dialog)  Indices=[13]  OutputSizes=1
  Selector2 : Selector  InputPortWidth=14  IndexOptions=Index vector (dialog)  Indices=[14]  OutputSizes=1
  Selector5 : Selector  InputPortWidth=14  IndexOptions=Index vector (dialog)  Indices=[1 2 3 4 5 6 7 8 9 10 11 12]  OutputSizes=1
  Out1 : Outport
  wires:
  In1/1 -> Selector5/1, Selector2/1, Selector1/1
  Selector5/1 -> Bus Creator/1  "Measurements"
  Bus Creator/1 -> Out1/1
  Selector1/1 -> Bus Creator/2  "FREQ"
  Selector2/1 -> Bus Creator/3  "FROC"

== system ng_pv_dynamic_dbus_p_4_ss_pmu/SS_PMU/Subsystem31/Subsystem ==
  In1 : Inport
  Bus Creator : BusCreator  Inputs=3
  Selector1 : Selector  InputPortWidth=14  IndexOptions=Index vector (dialog)  Indices=[13]  OutputSizes=1
  Selector2 : Selector  InputPortWidth=14  IndexOptions=Index vector (dialog)  Indices=[14]  OutputSizes=1
  Selector5 : Selector  InputPortWidth=14  IndexOptions=Index vector (dialog)  Indices=[1 2 3 4 5 6 7 8 9 10 11 12]  OutputSizes=1
  Out1 : Outport
  wires:
  In1/1 -> Selector5/1, Selector2/1, Selector1/1
  Selector5/1 -> Bus Creator/1  "Measurements"
  Bus Creator/1 -> Out1/1
  Selector1/1 -> Bus Creator/2  "FREQ"
  Selector2/1 -> Bus Creator/3  "FROC"

== system ng_pv_dynamic_dbus_p_4_ss_pmu/SS_PMU/Subsystem32/Subsystem ==
  In1 : Inport
  Bus Creator : BusCreator  Inputs=3
  Selector1 : Selector  InputPortWidth=14  IndexOptions=Index vector (dialog)  Indices=[13]  OutputSizes=1
  Selector2 : Selector  InputPortWidth=14  IndexOptions=Index vector (dialog)  Indices=[14]  OutputSizes=1
  Selector5 : Selector  InputPortWidth=14  IndexOptions=Index vector (dialog)  Indices=[1 2 3 4 5 6 7 8 9 10 11 12]  OutputSizes=1
  Out1 : Outport
  wires:
  In1/1 -> Selector5/1, Selector2/1, Selector1/1
  Selector5/1 -> Bus Creator/1  "Measurements"
  Bus Creator/1 -> Out1/1
  Selector1/1 -> Bus Creator/2  "FREQ"
  Selector2/1 -> Bus Creator/3  "FROC"

== system ng_pv_dynamic_dbus_p_4_ss_pmu/SS_PMU/Subsystem33/Subsystem ==
  In1 : Inport
  Bus Creator : BusCreator  Inputs=3
  Selector1 : Selector  InputPortWidth=14  IndexOptions=Index vector (dialog)  Indices=[13]  OutputSizes=1
  Selector2 : Selector  InputPortWidth=14  IndexOptions=Index vector (dialog)  Indices=[14]  OutputSizes=1
  Selector5 : Selector  InputPortWidth=14  IndexOptions=Index vector (dialog)  Indices=[1 2 3 4 5 6 7 8 9 10 11 12]  OutputSizes=1
  Out1 : Outport
  wires:
  In1/1 -> Selector5/1, Selector2/1, Selector1/1
  Selector5/1 -> Bus Creator/1  "Measurements"
  Bus Creator/1 -> Out1/1
  Selector1/1 -> Bus Creator/2  "FREQ"
  Selector2/1 -> Bus Creator/3  "FROC"

== system ng_pv_dynamic_dbus_p_4_ss_pmu/SS_PMU/Subsystem34/Subsystem ==
  In1 : Inport
  Bus Creator : BusCreator  Inputs=3
  Selector1 : Selector  InputPortWidth=14  IndexOptions=Index vector (dialog)  Indices=[13]  OutputSizes=1
  Selector2 : Selector  InputPortWidth=14  IndexOptions=Index vector (dialog)  Indices=[14]  OutputSizes=1
  Selector5 : Selector  InputPortWidth=14  IndexOptions=Index vector (dialog)  Indices=[1 2 3 4 5 6 7 8 9 10 11 12]  OutputSizes=1
  Out1 : Outport
  wires:
  In1/1 -> Selector5/1, Selector2/1, Selector1/1
  Selector5/1 -> Bus Creator/1  "Measurements"
  Bus Creator/1 -> Out1/1
  Selector1/1 -> Bus Creator/2  "FREQ"
  Selector2/1 -> Bus Creator/3  "FROC"

== system ng_pv_dynamic_dbus_p_4_ss_pmu/SS_PMU/Subsystem35/Subsystem ==
  In1 : Inport
  Bus Creator : BusCreator  Inputs=3
  Selector1 : Selector  InputPortWidth=14  IndexOptions=Index vector (dialog)  Indices=[13]  OutputSizes=1
  Selector2 : Selector  InputPortWidth=14  IndexOptions=Index vector (dialog)  Indices=[14]  OutputSizes=1
  Selector5 : Selector  InputPortWidth=14  IndexOptions=Index vector (dialog)  Indices=[1 2 3 4 5 6 7 8 9 10 11 12]  OutputSizes=1
  Out1 : Outport
  wires:
  In1/1 -> Selector5/1, Selector2/1, Selector1/1
  Selector5/1 -> Bus Creator/1  "Measurements"
  Bus Creator/1 -> Out1/1
  Selector1/1 -> Bus Creator/2  "FREQ"
  Selector2/1 -> Bus Creator/3  "FROC"

== system ng_pv_dynamic_dbus_p_4_ss_pmu/SS_PMU/Subsystem36/Subsystem ==
  In1 : Inport
  Bus Creator : BusCreator  Inputs=3
  Selector1 : Selector  InputPortWidth=14  IndexOptions=Index vector (dialog)  Indices=[13]  OutputSizes=1
  Selector2 : Selector  InputPortWidth=14  IndexOptions=Index vector (dialog)  Indices=[14]  OutputSizes=1
  Selector5 : Selector  InputPortWidth=14  IndexOptions=Index vector (dialog)  Indices=[1 2 3 4 5 6 7 8 9 10 11 12]  OutputSizes=1
  Out1 : Outport
  wires:
  In1/1 -> Selector5/1, Selector2/1, Selector1/1
  Selector5/1 -> Bus Creator/1  "Measurements"
  Bus Creator/1 -> Out1/1
  Selector1/1 -> Bus Creator/2  "FREQ"
  Selector2/1 -> Bus Creator/3  "FROC"

== system ng_pv_dynamic_dbus_p_4_ss_pmu/SS_PMU/Subsystem37/Subsystem ==
  In1 : Inport
  Bus Creator : BusCreator  Inputs=3
  Selector1 : Selector  InputPortWidth=14  IndexOptions=Index vector (dialog)  Indices=[13]  OutputSizes=1
  Selector2 : Selector  InputPortWidth=14  IndexOptions=Index vector (dialog)  Indices=[14]  OutputSizes=1
  Selector5 : Selector  InputPortWidth=14  IndexOptions=Index vector (dialog)  Indices=[1 2 3 4 5 6 7 8 9 10 11 12]  OutputSizes=1
  Out1 : Outport
  wires:
  In1/1 -> Selector5/1, Selector2/1, Selector1/1
  Selector5/1 -> Bus Creator/1  "Measurements"
  Bus Creator/1 -> Out1/1
  Selector1/1 -> Bus Creator/2  "FREQ"
  Selector2/1 -> Bus Creator/3  "FROC"

== system ng_pv_dynamic_dbus_p_4_ss_pmu/SS_PMU/Subsystem38/Subsystem ==
  In1 : Inport
  Bus Creator : BusCreator  Inputs=3
  Selector1 : Selector  InputPortWidth=14  IndexOptions=Index vector (dialog)  Indices=[13]  OutputSizes=1
  Selector2 : Selector  InputPortWidth=14  IndexOptions=Index vector (dialog)  Indices=[14]  OutputSizes=1
  Selector5 : Selector  InputPortWidth=14  IndexOptions=Index vector (dialog)  Indices=[1 2 3 4 5 6 7 8 9 10 11 12]  OutputSizes=1
  Out1 : Outport
  wires:
  In1/1 -> Selector5/1, Selector2/1, Selector1/1
  Selector5/1 -> Bus Creator/1  "Measurements"
  Bus Creator/1 -> Out1/1
  Selector1/1 -> Bus Creator/2  "FREQ"
  Selector2/1 -> Bus Creator/3  "FROC"

== system ng_pv_dynamic_dbus_p_4_ss_pmu/SS_PMU/Subsystem39/Subsystem ==
  In1 : Inport
  Bus Creator : BusCreator  Inputs=3
  Selector1 : Selector  InputPortWidth=14  IndexOptions=Index vector (dialog)  Indices=[13]  OutputSizes=1
  Selector2 : Selector  InputPortWidth=14  IndexOptions=Index vector (dialog)  Indices=[14]  OutputSizes=1
  Selector5 : Selector  InputPortWidth=14  IndexOptions=Index vector (dialog)  Indices=[1 2 3 4 5 6 7 8 9 10 11 12]  OutputSizes=1
  Out1 : Outport
  wires:
  In1/1 -> Selector5/1, Selector2/1, Selector1/1
  Selector5/1 -> Bus Creator/1  "Measurements"
  Bus Creator/1 -> Out1/1
  Selector1/1 -> Bus Creator/2  "FREQ"
  Selector2/1 -> Bus Creator/3  "FROC"

== system ng_pv_dynamic_dbus_p_4_ss_pmu/SS_PMU/Subsystem4/Subsystem ==
  Measurements1 : Inport
  Demux7 : Demux  Outputs=2
  Subsystem1 : Subsystem
  Phasors_Vabc : Outport
  Phasors_Iabc : Outport  Port=2
  Phasor_Freq : Outport  Port=3
  Phasor_DTFreq : Outport  Port=4
  wires:
  Measurements1/1 -> Subsystem1/1(Measurements)
  Subsystem1/2(Phasors_Freq) -> Phasor_Freq/1
  Subsystem1/3(Phasors_DTFreq) -> Phasor_DTFreq/1
  Demux7/2 -> Phasors_Iabc/1
  Demux7/1 -> Phasors_Vabc/1
  Subsystem1/1(Phasors_abc) -> Demux7/1

== system ng_pv_dynamic_dbus_p_4_ss_pmu/SS_PMU/Subsystem40/Subsystem ==
  In1 : Inport
  Bus Creator : BusCreator  Inputs=3
  Selector1 : Selector  InputPortWidth=14  IndexOptions=Index vector (dialog)  Indices=[13]  OutputSizes=1
  Selector2 : Selector  InputPortWidth=14  IndexOptions=Index vector (dialog)  Indices=[14]  OutputSizes=1
  Selector5 : Selector  InputPortWidth=14  IndexOptions=Index vector (dialog)  Indices=[1 2 3 4 5 6 7 8 9 10 11 12]  OutputSizes=1
  Out1 : Outport
  wires:
  In1/1 -> Selector5/1, Selector2/1, Selector1/1
  Selector5/1 -> Bus Creator/1  "Measurements"
  Bus Creator/1 -> Out1/1
  Selector1/1 -> Bus Creator/2  "FREQ"
  Selector2/1 -> Bus Creator/3  "FROC"

== system ng_pv_dynamic_dbus_p_4_ss_pmu/SS_PMU/Subsystem41/Subsystem ==
  In1 : Inport
  Bus Creator : BusCreator  Inputs=3
  Selector1 : Selector  InputPortWidth=14  IndexOptions=Index vector (dialog)  Indices=[13]  OutputSizes=1
  Selector2 : Selector  InputPortWidth=14  IndexOptions=Index vector (dialog)  Indices=[14]  OutputSizes=1
  Selector5 : Selector  InputPortWidth=14  IndexOptions=Index vector (dialog)  Indices=[1 2 3 4 5 6 7 8 9 10 11 12]  OutputSizes=1
  Out1 : Outport
  wires:
  In1/1 -> Selector5/1, Selector2/1, Selector1/1
  Selector5/1 -> Bus Creator/1  "Measurements"
  Bus Creator/1 -> Out1/1
  Selector1/1 -> Bus Creator/2  "FREQ"
  Selector2/1 -> Bus Creator/3  "FROC"

== system ng_pv_dynamic_dbus_p_4_ss_pmu/SS_PMU/Subsystem42/Subsystem ==
  In1 : Inport
  Bus Creator : BusCreator  Inputs=3
  Selector1 : Selector  InputPortWidth=14  IndexOptions=Index vector (dialog)  Indices=[13]  OutputSizes=1
  Selector2 : Selector  InputPortWidth=14  IndexOptions=Index vector (dialog)  Indices=[14]  OutputSizes=1
  Selector5 : Selector  InputPortWidth=14  IndexOptions=Index vector (dialog)  Indices=[1 2 3 4 5 6 7 8 9 10 11 12]  OutputSizes=1
  Out1 : Outport
  wires:
  In1/1 -> Selector5/1, Selector2/1, Selector1/1
  Selector5/1 -> Bus Creator/1  "Measurements"
  Bus Creator/1 -> Out1/1
  Selector1/1 -> Bus Creator/2  "FREQ"
  Selector2/1 -> Bus Creator/3  "FROC"

== system ng_pv_dynamic_dbus_p_4_ss_pmu/SS_PMU/Subsystem43/Subsystem ==
  In1 : Inport
  Bus Creator : BusCreator  Inputs=3
  Selector1 : Selector  InputPortWidth=14  IndexOptions=Index vector (dialog)  Indices=[13]  OutputSizes=1
  Selector2 : Selector  InputPortWidth=14  IndexOptions=Index vector (dialog)  Indices=[14]  OutputSizes=1
  Selector5 : Selector  InputPortWidth=14  IndexOptions=Index vector (dialog)  Indices=[1 2 3 4 5 6 7 8 9 10 11 12]  OutputSizes=1
  Out1 : Outport
  wires:
  In1/1 -> Selector5/1, Selector2/1, Selector1/1
  Selector5/1 -> Bus Creator/1  "Measurements"
  Bus Creator/1 -> Out1/1
  Selector1/1 -> Bus Creator/2  "FREQ"
  Selector2/1 -> Bus Creator/3  "FROC"

== system ng_pv_dynamic_dbus_p_4_ss_pmu/SS_PMU/Subsystem44/Subsystem ==
  In1 : Inport
  Bus Creator : BusCreator  Inputs=3
  Selector1 : Selector  InputPortWidth=14  IndexOptions=Index vector (dialog)  Indices=[13]  OutputSizes=1
  Selector2 : Selector  InputPortWidth=14  IndexOptions=Index vector (dialog)  Indices=[14]  OutputSizes=1
  Selector5 : Selector  InputPortWidth=14  IndexOptions=Index vector (dialog)  Indices=[1 2 3 4 5 6 7 8 9 10 11 12]  OutputSizes=1
  Out1 : Outport
  wires:
  In1/1 -> Selector5/1, Selector2/1, Selector1/1
  Selector5/1 -> Bus Creator/1  "Measurements"
  Bus Creator/1 -> Out1/1
  Selector1/1 -> Bus Creator/2  "FREQ"
  Selector2/1 -> Bus Creator/3  "FROC"

== system ng_pv_dynamic_dbus_p_4_ss_pmu/SS_PMU/Subsystem5/Subsystem ==
  Measurements1 : Inport
  Demux7 : Demux  Outputs=2
  Subsystem1 : Subsystem
  Phasors_Vabc : Outport
  Phasors_Iabc : Outport  Port=2
  Phasor_Freq : Outport  Port=3
  Phasor_DTFreq : Outport  Port=4
  wires:
  Measurements1/1 -> Subsystem1/1(Measurements)
  Subsystem1/2(Phasors_Freq) -> Phasor_Freq/1
  Subsystem1/3(Phasors_DTFreq) -> Phasor_DTFreq/1
  Demux7/2 -> Phasors_Iabc/1
  Demux7/1 -> Phasors_Vabc/1
  Subsystem1/1(Phasors_abc) -> Demux7/1

== system ng_pv_dynamic_dbus_p_4_ss_pmu/SS_PMU/Subsystem6/Subsystem ==
  Measurements1 : Inport
  Demux7 : Demux  Outputs=2
  Subsystem1 : Subsystem
  Phasors_Vabc : Outport
  Phasors_Iabc : Outport  Port=2
  Phasor_Freq : Outport  Port=3
  Phasor_DTFreq : Outport  Port=4
  wires:
  Measurements1/1 -> Subsystem1/1(Measurements)
  Subsystem1/2(Phasors_Freq) -> Phasor_Freq/1
  Subsystem1/3(Phasors_DTFreq) -> Phasor_DTFreq/1
  Demux7/2 -> Phasors_Iabc/1
  Demux7/1 -> Phasors_Vabc/1
  Subsystem1/1(Phasors_abc) -> Demux7/1

== system ng_pv_dynamic_dbus_p_4_ss_pmu/SS_PMU/Subsystem7/Subsystem ==
  Measurements1 : Inport
  Demux7 : Demux  Outputs=2
  Subsystem1 : Subsystem
  Phasors_Vabc : Outport
  Phasors_Iabc : Outport  Port=2
  Phasor_Freq : Outport  Port=3
  Phasor_DTFreq : Outport  Port=4
  wires:
  Measurements1/1 -> Subsystem1/1(Measurements)
  Subsystem1/2(Phasors_Freq) -> Phasor_Freq/1
  Subsystem1/3(Phasors_DTFreq) -> Phasor_DTFreq/1
  Demux7/2 -> Phasors_Iabc/1
  Demux7/1 -> Phasors_Vabc/1
  Subsystem1/1(Phasors_abc) -> Demux7/1

== system ng_pv_dynamic_dbus_p_4_ss_pmu/SS_PMU/Subsystem8/Subsystem ==
  Measurements1 : Inport
  Demux7 : Demux  Outputs=2
  Subsystem1 : Subsystem
  Phasors_Vabc : Outport
  Phasors_Iabc : Outport  Port=2
  Phasor_Freq : Outport  Port=3
  Phasor_DTFreq : Outport  Port=4
  wires:
  Measurements1/1 -> Subsystem1/1(Measurements)
  Subsystem1/2(Phasors_Freq) -> Phasor_Freq/1
  Subsystem1/3(Phasors_DTFreq) -> Phasor_DTFreq/1
  Demux7/2 -> Phasors_Iabc/1
  Demux7/1 -> Phasors_Vabc/1
  Subsystem1/1(Phasors_abc) -> Demux7/1

== system ng_pv_dynamic_dbus_p_4_ss_pmu/SS_PMU/Subsystem9/Subsystem ==
  Measurements1 : Inport
  Demux7 : Demux  Outputs=2
  Subsystem1 : Subsystem
  Phasors_Vabc : Outport
  Phasors_Iabc : Outport  Port=2
  Phasor_Freq : Outport  Port=3
  Phasor_DTFreq : Outport  Port=4
  wires:
  Measurements1/1 -> Subsystem1/1(Measurements)
  Subsystem1/2(Phasors_Freq) -> Phasor_Freq/1
  Subsystem1/3(Phasors_DTFreq) -> Phasor_DTFreq/1
  Demux7/2 -> Phasors_Iabc/1
  Demux7/1 -> Phasors_Vabc/1
  Subsystem1/1(Phasors_abc) -> Demux7/1

== system ng_pv_dynamic_dbus_p_4_ss_pmu/SS_PMU/rtlab_send_subsystem/Subsystem1 ==
  In1 : Inport
  Mux : Mux  Inputs=1
  Send1 : opal_lib/Communication/OpSendToNT  Acqu_group=1
  wires:
  Mux/1 -> Send1/1
  In1/1 -> Mux/1

== system ng_pv_dynamic_dbus_p_4_ss_pmu/SS_PMU/zzzOpComm/busStruct ==
  In1 : Inport
  In2 : Inport  Port=2
  In3 : Inport  Port=3
  Sub1 : Subsystem
  Sub2 : Subsystem
  Sub3 : Subsystem
  Out1 : Outport
  Out2 : Outport  Port=2
  Out3 : Outport  Port=3
  wires:
  Sub3/1(out) -> Out3/1
  In3/1 -> Sub3/1(in)
  Sub2/1(out) -> Out2/1
  In2/1 -> Sub2/1(in)
  Sub1/1(goto_signal1) -> Out1/1
  In1/1 -> Sub1/1(from_signal1)

== system ng_pv_dynamic_dbus_p_4_ss_pmu/SS_PMU/Subsystem1/Subsystem/Subsystem1 ==
  Measurements : Inport
  Degree to radian1 : Subsystem
  Mux1 : Mux
  Selector5 : Selector  InputPortWidth=12  IndexOptions=Index vector (dialog)  Indices=[1 3 5]  OutputSizes=1
  Selector6 : Selector  InputPortWidth=12  IndexOptions=Index vector (dialog)  Indices=[7 9 11]  OutputSizes=1
  Selector7 : Selector  InputPortWidth=6  IndexOptions=Index vector (dialog)  Indices=[1 2 3]  OutputSizes=1
  Selector8 : Selector  InputPortWidth=6  IndexOptions=Index vector (dialog)  Indices=[4 5 6]  OutputSizes=1
  Selector9 : Selector  InputPortWidth=12  IndexOptions=Index vector (dialog)  Indices=[2 4 6 8 10 12]  OutputSizes=1
  Subsystem : Subsystem
  Phasors_abc : Outport
  Phasors_Freq : Outport  Port=2
  Phasors_DTFreq : Outport  Port=3
  wires:
  Subsystem/2(Phasors_freq) -> Phasors_Freq/1
  Subsystem/3(Phasors_dtfreq1) -> Phasors_DTFreq/1
  Selector5/1 -> Mux1/1
  Mux1/1 -> Phasors_abc/1
  Selector7/1 -> Mux1/2
  Subsystem/1(Phasors_60Hz) -> Selector5/1, Selector6/1, Selector9/1
  Selector8/1 -> Mux1/4
  Selector6/1 -> Mux1/3
  Measurements/1 -> Subsystem/1(Measurements1)
  Selector9/1 -> Degree to radian1/1(Degree)
  Degree to radian1/1(Radian) -> Selector7/1, Selector8/1

== system ng_pv_dynamic_dbus_p_4_ss_pmu/SS_PMU/Subsystem10/Subsystem/Subsystem1 ==
  Measurements : Inport
  Degree to radian1 : Subsystem
  Mux1 : Mux
  Selector5 : Selector  InputPortWidth=12  IndexOptions=Index vector (dialog)  Indices=[1 3 5]  OutputSizes=1
  Selector6 : Selector  InputPortWidth=12  IndexOptions=Index vector (dialog)  Indices=[7 9 11]  OutputSizes=1
  Selector7 : Selector  InputPortWidth=6  IndexOptions=Index vector (dialog)  Indices=[1 2 3]  OutputSizes=1
  Selector8 : Selector  InputPortWidth=6  IndexOptions=Index vector (dialog)  Indices=[4 5 6]  OutputSizes=1
  Selector9 : Selector  InputPortWidth=12  IndexOptions=Index vector (dialog)  Indices=[2 4 6 8 10 12]  OutputSizes=1
  Subsystem : Subsystem
  Phasors_abc : Outport
  Phasors_Freq : Outport  Port=2
  Phasors_DTFreq : Outport  Port=3
  wires:
  Subsystem/2(Phasors_freq) -> Phasors_Freq/1
  Subsystem/3(Phasors_dtfreq1) -> Phasors_DTFreq/1
  Selector5/1 -> Mux1/1
  Mux1/1 -> Phasors_abc/1
  Selector7/1 -> Mux1/2
  Subsystem/1(Phasors_60Hz) -> Selector5/1, Selector6/1, Selector9/1
  Selector8/1 -> Mux1/4
  Selector6/1 -> Mux1/3
  Measurements/1 -> Subsystem/1(Measurements1)
  Selector9/1 -> Degree to radian1/1(Degree)
  Degree to radian1/1(Radian) -> Selector7/1, Selector8/1

== system ng_pv_dynamic_dbus_p_4_ss_pmu/SS_PMU/Subsystem11/Subsystem/Subsystem1 ==
  Measurements : Inport
  Degree to radian1 : Subsystem
  Mux1 : Mux
  Selector5 : Selector  InputPortWidth=12  IndexOptions=Index vector (dialog)  Indices=[1 3 5]  OutputSizes=1
  Selector6 : Selector  InputPortWidth=12  IndexOptions=Index vector (dialog)  Indices=[7 9 11]  OutputSizes=1
  Selector7 : Selector  InputPortWidth=6  IndexOptions=Index vector (dialog)  Indices=[1 2 3]  OutputSizes=1
  Selector8 : Selector  InputPortWidth=6  IndexOptions=Index vector (dialog)  Indices=[4 5 6]  OutputSizes=1
  Selector9 : Selector  InputPortWidth=12  IndexOptions=Index vector (dialog)  Indices=[2 4 6 8 10 12]  OutputSizes=1
  Subsystem : Subsystem
  Phasors_abc : Outport
  Phasors_Freq : Outport  Port=2
  Phasors_DTFreq : Outport  Port=3
  wires:
  Subsystem/2(Phasors_freq) -> Phasors_Freq/1
  Subsystem/3(Phasors_dtfreq1) -> Phasors_DTFreq/1
  Selector5/1 -> Mux1/1
  Mux1/1 -> Phasors_abc/1
  Selector7/1 -> Mux1/2
  Subsystem/1(Phasors_60Hz) -> Selector5/1, Selector6/1, Selector9/1
  Selector8/1 -> Mux1/4
  Selector6/1 -> Mux1/3
  Measurements/1 -> Subsystem/1(Measurements1)
  Selector9/1 -> Degree to radian1/1(Degree)
  Degree to radian1/1(Radian) -> Selector7/1, Selector8/1

== system ng_pv_dynamic_dbus_p_4_ss_pmu/SS_PMU/Subsystem12/Subsystem/Subsystem1 ==
  Measurements : Inport
  Degree to radian1 : Subsystem
  Mux1 : Mux
  Selector5 : Selector  InputPortWidth=12  IndexOptions=Index vector (dialog)  Indices=[1 3 5]  OutputSizes=1
  Selector6 : Selector  InputPortWidth=12  IndexOptions=Index vector (dialog)  Indices=[7 9 11]  OutputSizes=1
  Selector7 : Selector  InputPortWidth=6  IndexOptions=Index vector (dialog)  Indices=[1 2 3]  OutputSizes=1
  Selector8 : Selector  InputPortWidth=6  IndexOptions=Index vector (dialog)  Indices=[4 5 6]  OutputSizes=1
  Selector9 : Selector  InputPortWidth=12  IndexOptions=Index vector (dialog)  Indices=[2 4 6 8 10 12]  OutputSizes=1
  Subsystem : Subsystem
  Phasors_abc : Outport
  Phasors_Freq : Outport  Port=2
  Phasors_DTFreq : Outport  Port=3
  wires:
  Subsystem/2(Phasors_freq) -> Phasors_Freq/1
  Subsystem/3(Phasors_dtfreq1) -> Phasors_DTFreq/1
  Selector5/1 -> Mux1/1
  Mux1/1 -> Phasors_abc/1
  Selector7/1 -> Mux1/2
  Subsystem/1(Phasors_60Hz) -> Selector5/1, Selector6/1, Selector9/1
  Selector8/1 -> Mux1/4
  Selector6/1 -> Mux1/3
  Measurements/1 -> Subsystem/1(Measurements1)
  Selector9/1 -> Degree to radian1/1(Degree)
  Degree to radian1/1(Radian) -> Selector7/1, Selector8/1
